simulink library "VsrLibDriver"  (R2019b)
settings: Solver=VariableStepAuto  StartTime=0.0  StopTime=10.0  RelTol=1e-3
undefined symbols (not defined in the file): ChassisVehMass, EnvGravCnst
libraries: $bdroot x1
settings Model: Creator=9bt  LastModifiedBy=4qz

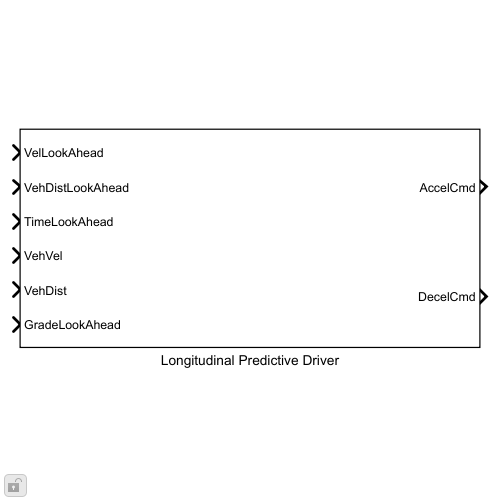
[thumbnail: Simulink's stored preview of the top-level diagram]
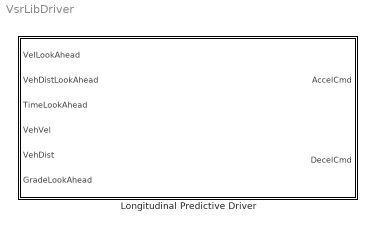
== system VsrLibDriver ==
  Longitudinal Predictive Driver : Subsystem  mask{VehMass=ChassisVehMass, aR=20000, bR=1, cR=4, MaxAccelFrcSpdBpts=[ 10, 100 ], MaxAccelFrcTbl=[ 150000, 150000 ], AccelPdlBpts=[ 0, 1 ], AccelPdlTbl=[ 0, 1 ], BrakePdlBpts=[ 0, 1 ], BrakeFrcTbl=[ 0, 180000 ], SmoothTimeAvg=.5, VelThresh=.5, PdlRateLimitWeight=.1, DistOptWeight=.2, NumOptimIters=20, g=EnvGravCnst}
      mask prompts: VehMass "Vehicle mass, VehMass [kg]:"; aR "Rolling resistance coefficient, aR [N]:"; bR "Rolling and driveline resistance coefficient, bR [N*s/m]:"; cR "Aerodynamic drag coefficient, cR [N*s^2/m^2]:"; MaxAccelFrcSpdBpts "Max acceleration force speed breakpoints, MaxAccelFrcSpdBpts [m/s]:"; MaxAccelFrcTbl "Max acceleration force table, MaxAccelFrcTbl [N]:"; AccelPdlBpts "Accelerator pedal position breakpoints, AccelPdlBpts []:"; AccelPdlTbl "Accelerator pedal position table, AccelPdlTbl []:"; BrakePdlBpts "Brake pedal position breakpoints, BrakePdlBpts []:"; BrakeFrcTbl "Brake force table, BrakeFrcTbl [N]:"; SmoothTimeAvg "Time average smoothing time, SmoothTimeAvg [s]:"; VelThresh "Velocity threshold for calculating losses, VelThresh [m/s]:"; PdlRateLimitWeight "Pedal rate limit weight, PdlRateLimitWeight []:"; DistOptWeight "Distance optimization weight, DistOptWeight []:"; NumOptimIters "Number of optimization iterations, NumOptimIters []:"; g "Gravitational constant, g [m/s^2]:"
      mask TypeOptions VehMass: Longitudinal Predictive Driver/VehMass
      mask TypeOptions aR: Longitudinal Predictive Driver/aR
      mask TypeOptions bR: Longitudinal Predictive Driver/bR
      mask TypeOptions cR: Longitudinal Predictive Driver/cR
      mask TypeOptions MaxAccelFrcSpdBpts: Longitudinal Predictive Driver/MaxAccelFrcSpdBpts
      mask TypeOptions MaxAccelFrcTbl: Longitudinal Predictive Driver/MaxAccelFrcTbl
      mask TypeOptions AccelPdlBpts: Longitudinal Predictive Driver/AccelPdlBpts
      mask TypeOptions AccelPdlTbl: Longitudinal Predictive Driver/AccelPdlTbl
      mask TypeOptions BrakePdlBpts: Longitudinal Predictive Driver/BrakePdlBpts
      mask TypeOptions BrakeFrcTbl: Longitudinal Predictive Driver/BrakeFrcTbl
      mask TypeOptions VelThresh: Longitudinal Predictive Driver/VelThresh
      mask TypeOptions PdlRateLimitWeight: Longitudinal Predictive Driver/PdlRateLimitWeight
      mask TypeOptions DistOptWeight: Longitudinal Predictive Driver/DistOptWeight
      mask TypeOptions NumOptimIters: Longitudinal Predictive Driver/NumOptimIters
      mask TypeOptions g: Longitudinal Predictive Driver/g

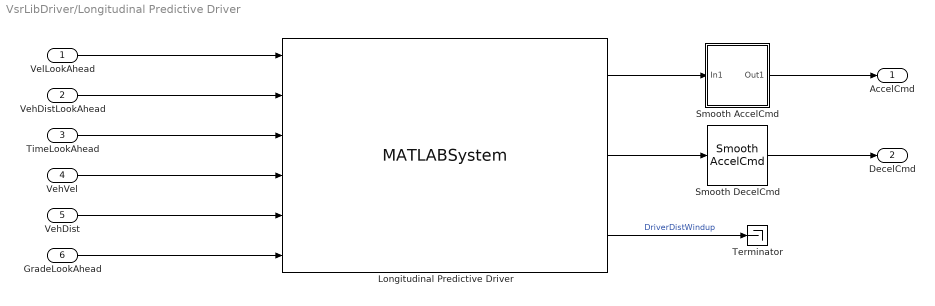
== system VsrLibDriver/Longitudinal Predictive Driver ==
  VelLookAhead : Inport  Unit=m/s
  VehDistLookAhead : Inport  Port=2  Unit=s
  TimeLookAhead : Inport  Port=3  Unit=s
  VehVel : Inport  Port=4  Unit=m/s
  VehDist : Inport  Port=5  Unit=m
  GradeLookAhead : Inport  Port=6  Unit=rad
  Longitudinal Predictive Driver : MATLABSystem  System=vsr.mdl.driver.LongitudinalPredDriver  VehMass=VehMass  aR=aR  bR=bR  cR=cR  g=g  MaxAccelFrcSpdBpts=MaxAccelFrcSpdBpts  MaxAccelFrcTbl=MaxAccelFrcTbl  AccelPdlBpts=AccelPdlBpts  AccelPdlTbl=AccelPdlTbl  BrakePdlBpts=BrakePdlBpts  BrakeFrcTbl=BrakeFrcTbl  VelThresh=VelThresh  DistOptWeight=DistOptWeight  PdlRateLimitWeight=PdlRateLimitWeight  NumOptimIters=NumOptimIters  SimulateUsing=Code generation
      mask Type: vsr.mdl.driver.LongitudinalPredDriver
      mask Display:
      | disp('LongitudinalPredDriver');
      | port_label('input',1,'VelLookAhead');
      | port_label('input',2,'VehDistLookAhead');
      | port_label('input',3,'TimeLookAhead');
      | port_label('input',4,'VehVel');
      | port_label('input',5,'VehDist');
      | port_label('input',6,'GradeLookAhead');
      | port_label('output',1,'AccelCmd');
      | port_label('output',2,'DecelCmd');
      | port_label('output',3,'DistWindupOut');
  Smooth AccelCmd : Subsystem
  Smooth DecelCmd : $bdroot/Longitudinal Predictive Driver/Smooth AccelCmd  SystemSampleTime=-1  Latency=0  AutoFrameSizeCalculation=off
  Terminator : Terminator
  AccelCmd : Outport
  DecelCmd : Outport  Port=2
  wires:
  Longitudinal Predictive Driver/3 -> Terminator/1  "DriverDistWindup"
  VelLookAhead/1 -> Longitudinal Predictive Driver/1
  TimeLookAhead/1 -> Longitudinal Predictive Driver/3
  GradeLookAhead/1 -> Longitudinal Predictive Driver/6
  VehVel/1 -> Longitudinal Predictive Driver/4
  VehDistLookAhead/1 -> Longitudinal Predictive Driver/2
  VehDist/1 -> Longitudinal Predictive Driver/5
  Longitudinal Predictive Driver/1 -> Smooth AccelCmd/1(In1)
  Smooth AccelCmd/1(Out1) -> AccelCmd/1
  Smooth DecelCmd/1 -> DecelCmd/1
  Longitudinal Predictive Driver/2 -> Smooth DecelCmd/1

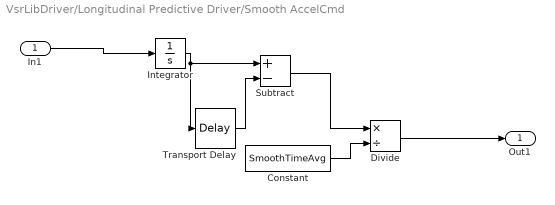
== system VsrLibDriver/Longitudinal Predictive Driver/Smooth AccelCmd ==
  In1 : Inport
  Constant : Constant  Value=SmoothTimeAvg
  Divide : Product  Inputs=*/
  Integrator : Integrator
  Subtract : Sum  Inputs=+-
  Transport Delay : TransportDelay  DelayTime=SmoothTimeAvg
  Out1 : Outport
  wires:
  In1/1 -> Integrator/1
  Subtract/1 -> Divide/1
  Constant/1 -> Divide/2
  Divide/1 -> Out1/1
  Integrator/1 -> Subtract/1, Transport Delay/1
  Transport Delay/1 -> Subtract/2
